simulink model "PID_diskret_optim1"  (R2021b)
settings: Solver=FixedStepAuto  StartTime=0.0  StopTime=0.1  FixedStep=1e-6  MaxStep=0.024  RelTol=1e-3
values from neighbouring files (symbols this model uses):
  K = ku*1/ke    (= 62.4349635796)    [tf_dpt_pr_6.m]
  Kd = 0.007    [tf_dpt_pr_6.m]
  Ki = 32.51    [tf_dpt_pr_6.m]
  Kp = 0.319    [tf_dpt_pr_6.m]
  N = 90780    [tf_dpt_pr_6.m]
  T1 = Te    (= 0.00682352941176)    [tf_dpt_pr_6.m]
  T2 = 1/(k1*k2*ke)    (= 0.0387062371254)    [tf_dpt_pr_6.m]
  Ts = 1e-6    (= 1e-06)    [tf_dpt_pr_6.m]
undefined symbols (not defined in the file or in its folder): dend, DiscIntNeverNeededParam, numd
libraries: checkpacklib x1
settings Model: Creator=Admin  LastModifiedBy=79159
settings SolverCC: AlgebraicLoopSolver=TrustRegion
settings DebuggingCC: SFMachineParentedDataDiag=warning

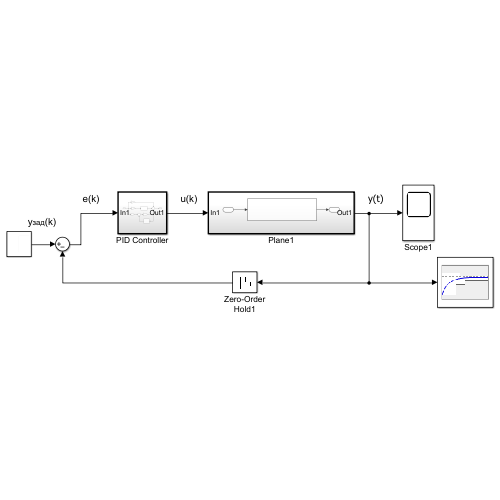
[thumbnail: Simulink's stored preview of the top-level diagram]
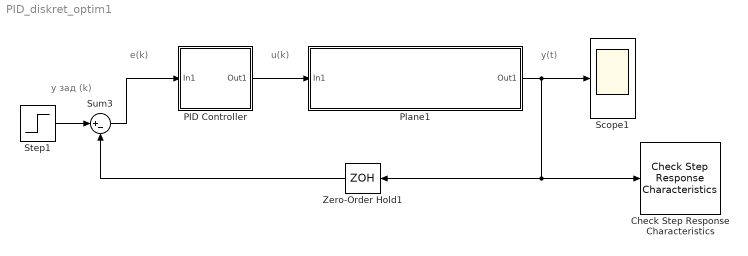
== system PID_diskret_optim1 ==
  note: y(t)
  note: u(k)
  note: y зад (k)
  note: e(k)
  Check Step Response Characteristics : checkpacklib/Check Step Response  Characteristics  InstantiateOnLoad=on  enabled=on  stopWhenAssertionFail=off  export=off  ViewDlgPos=[]  OpenViewOnLoad=off  LaunchViewOnOpen=off  TimeUnits=seconds  EnableStepResponseBound=on  InitialValue=0  FinalValue=1  StepTime=0  RiseTime=0.01  PercentRise=80  SettlingTime=0.04  PercentSettling=1  PercentOvershoot=5  PercentUndershoot=1
      settings: SourceProductBaseCode=CT,ID,MT,SO
  PID Controller : Subsystem  TreatAsAtomicUnit=on
  Plane1 : Subsystem  TreatAsAtomicUnit=on
  Scope1 : Scope
  Step1 : Step  Time=0  SampleTime=Ts  mask(DiscretizedSource){}
      mask init:
      | %zoh
  Sum3 : Sum  Inputs=|+-
  Zero-Order Hold1 : ZeroOrderHold  SampleTime=Ts
  wires:
  Step1/1 -> Sum3/1
  Zero-Order Hold1/1 -> Sum3/2
  Sum3/1 -> PID Controller/1(In1)
  Plane1/1(Out1) -> Scope1/1, Zero-Order Hold1/1, Check Step Response Characteristics/1
  PID Controller/1(Out1) -> Plane1/1(In1)

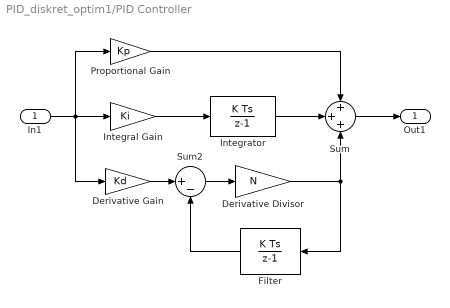
== system PID_diskret_optim1/PID Controller ==
  In1 : Inport
  Derivative Divisor : Gain  Gain=N  SaturateOnIntegerOverflow=on  OutDataTypeStr=Inherit: Same as input  ParamDataTypeStr=Inherit: Same as input
  Derivative Gain : Gain  Gain=Kd  SaturateOnIntegerOverflow=on  OutDataTypeStr=Inherit: Same as input  ParamDataTypeStr=Inherit: Same as input
  Filter : DiscreteIntegrator  SampleTime=Ts  ICPrevOutput=DiscIntNeverNeededParam  ICPrevScaledInput=DiscIntNeverNeededParam  mask(DiscretizedDiscreteIntegrator){}
      mask init:
      | %zoh
  Integral Gain : Gain  Gain=Ki  SaturateOnIntegerOverflow=on  OutDataTypeStr=Inherit: Same as input  ParamDataTypeStr=Inherit: Same as input
  Integrator : DiscreteIntegrator  SampleTime=Ts  ICPrevOutput=DiscIntNeverNeededParam  ICPrevScaledInput=DiscIntNeverNeededParam  mask(DiscretizedDiscreteIntegrator){}
      mask init:
      | %zoh
  Proportional Gain : Gain  Gain=Kp  SaturateOnIntegerOverflow=on  OutDataTypeStr=Inherit: Same as input  ParamDataTypeStr=Inherit: Same as input
  Sum : Sum  Inputs=+++  InputSameDT=on  SaturateOnIntegerOverflow=on  OutDataTypeStr=Inherit: Same as first input
  Sum2 : Sum  Inputs=|+-  InputSameDT=on  SaturateOnIntegerOverflow=on  OutDataTypeStr=Inherit: Same as first input
  Out1 : Outport
  wires:
  In1/1 -> Integral Gain/1, Proportional Gain/1, Derivative Gain/1
  Derivative Gain/1 -> Sum2/1
  Integral Gain/1 -> Integrator/1
  Filter/1 -> Sum2/2
  Integrator/1 -> Sum/2
  Sum2/1 -> Derivative Divisor/1
  Derivative Divisor/1 -> Filter/1, Sum/3
  Proportional Gain/1 -> Sum/1
  Sum/1 -> Out1/1

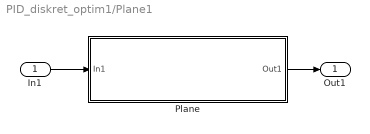
== system PID_diskret_optim1/Plane1 ==
  In1 : Inport
  Plane : Subsystem  mask(DiscretizedTransferFcn){Numerator=[K], Denominator=[T1*T2 T2 1], AbsTol=auto, SampleTime=Ts, method=zoh, Wc=0}
      mask prompts: Numerator "Numerator (enter in s-domain:)"; Denominator "Denominator (enter in s-domain:)"; AbsTol "Absolute tolerance:"; SampleTime "Sample time:"; Wc "Critical Frequency (Hz):"
      mask help: Continuous mask uses c2d to transform parameters onto the Discrete Transfer function block inside.
      mask init:
      | st=SampleTime;
      | if length(st)>1
      |     st=SampleTime(1);
      | end
      | if(st>0)
      |     [numd,dend] = sldiscutil('disctransferfcn',{st,method,Wc,Numerator,Denominator});
      | end	
      | s = get_param(gcb,'maskvalues');
      | nums = s{1};
      | dens = s{2};
      | %numc = eval(nums);
      | %denc = eval(dens);
      | sldiscutil('inittfmask', st);
      | if(st==0)
      | set_param([gcb '/Transfer Fcn'], 'AbsoluteTolerance', AbsTol);
      | end
      mask TypeOptions method: zoh | foh | tustin | prewarp | matched
      mask Callback method: hidecrit
      mask Display:
      | dpoly(nums,dens)
      | text( 0.5, 1.0, method, 'verticalAlignment','top','horizontalAlignment', 'center')
  Out1 : Outport
  wires:
  Plane/1(Out1) -> Out1/1
  In1/1 -> Plane/1(In1)

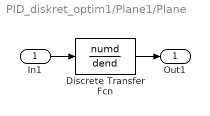
== system PID_diskret_optim1/Plane1/Plane ==
  In1 : Inport
  Discrete Transfer Fcn : DiscreteTransferFcn  Numerator=numd  Denominator=dend  SampleTime=SampleTime
  Out1 : Outport
  wires:
  In1/1 -> Discrete Transfer Fcn/1
  Discrete Transfer Fcn/1 -> Out1/1
